simulink library "TurnLightMode_Control"  (R2023a)
settings: Solver=VariableStepAuto  StartTime=0.0  StopTime=10.0  RelTol=1e-3
settings Model: Creator=19856  LastModifiedBy=19856

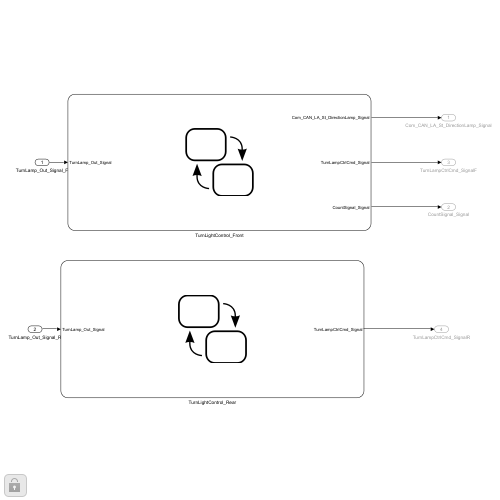
[thumbnail: Simulink's stored preview of the top-level diagram]
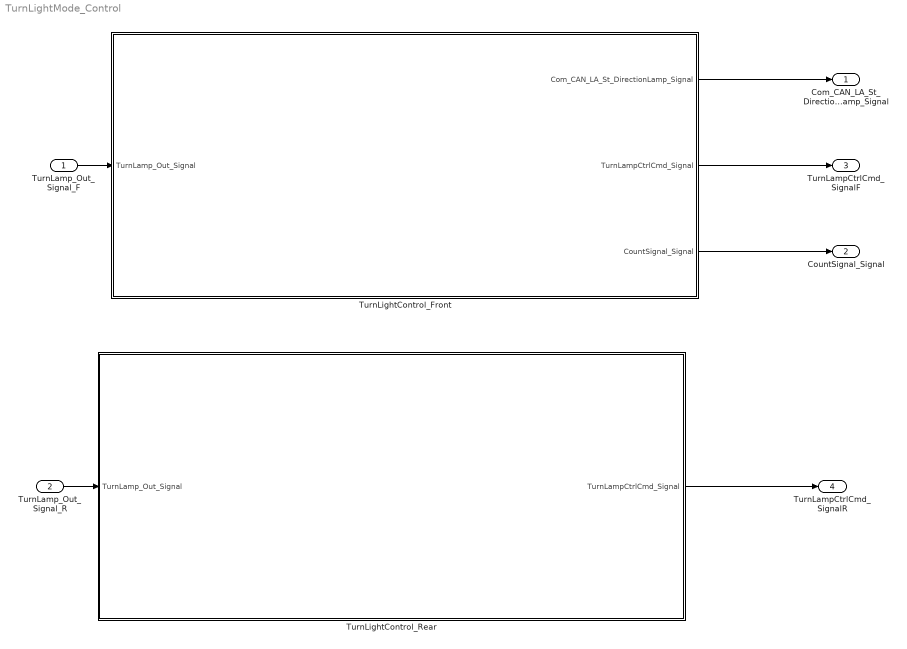
== system TurnLightMode_Control ==
  TurnLamp_Out_Signal_F : Inport
  TurnLamp_Out_Signal_R : Inport  Port=2
  TurnLightControl_Front : Stateflow chart  TreatAsAtomicUnit=on
  TurnLightControl_Rear : Stateflow chart  TreatAsAtomicUnit=on
  Com_CAN_LA_St_DirectionLamp_Signal : Outport
      settings: EnsureOutportIsVirtual=on
  CountSignal_Signal : Outport  Port=2
      settings: EnsureOutportIsVirtual=on
  TurnLampCtrlCmd_SignalF : Outport  Port=3
      settings: EnsureOutportIsVirtual=on
  TurnLampCtrlCmd_SignalR : Outport  Port=4
      settings: EnsureOutportIsVirtual=on
  wires:
  TurnLightControl_Front/2(TurnLampCtrlCmd_Signal) -> TurnLampCtrlCmd_SignalF/1
  TurnLightControl_Front/3(CountSignal_Signal) -> CountSignal_Signal/1
  TurnLamp_Out_Signal_F/1 -> TurnLightControl_Front/1(TurnLamp_Out_Signal)
  TurnLightControl_Front/1(Com_CAN_LA_St_DirectionLamp_Signal) -> Com_CAN_LA_St_DirectionLamp_Signal/1
  TurnLamp_Out_Signal_R/1 -> TurnLightControl_Rear/1(TurnLamp_Out_Signal)
  TurnLightControl_Rear/1(TurnLampCtrlCmd_Signal) -> TurnLampCtrlCmd_SignalR/1

== stateflow chart TurnLightMode_Control/TurnLightControl_Rear ==
  state IDLE
    en:
    TurnLampCtrlCmd_Signal=OFF;
  state LONG
    en:
    CountSignal_Signal=0;
    state OFF
      en:
      TurnLampCtrlCmd_Signal=OFF;
      ex:
      CountSignal_Signal++;
    state ON_
      en:
      TurnLampCtrlCmd_Signal=ON;
    (default) -> LONG.ON_
    LONG.ON_ -> LONG.OFF : [after(400,msec)]
    LONG.OFF -> LONG.ON_ : [after(400,msec)]
  state THREE
    en:
    CountSignal_Signal=0;
    state OFF
      en:
      TurnLampCtrlCmd_Signal=OFF;
      ex:
      CountSignal_Signal++;
    state ON_
      en:
      TurnLampCtrlCmd_Signal=ON;
    (default) -> THREE.ON_
    THREE.ON_ -> THREE.OFF : [after(200,msec)]
    THREE.OFF -> THREE.ON_ : [after(200,msec)]
  (default) -> IDLE
  IDLE -> LONG [order 2] : [TurnLamp_Out_Signal==MODE_LONG||...
      | TurnLamp_Out_Signal==MODE_THREE]
  LONG -> IDLE [order 2] : [TurnLamp_Out_Signal==MODE_THREE&&...
      | CountSignal_Signal==3]
  LONG -> IDLE [order 1] : [hasChangedFrom(TurnLamp_Out_Signal,MODE_LONG)]
  IDLE -> THREE [order 1] : [TurnLamp_Out_Signal==MODE_DOUBLE]
  THREE -> IDLE : [TurnLamp_Out_Signal!=MODE_DOUBLE]
  data: TurnLamp_Out_Signal input uint8; TurnLampCtrlCmd_Signal output uint8; CountSignal_Signal local uint8 =0; MODE_LONG constant uint8 =2; MODE_THREE constant uint8 =1; OFF constant uint8 =0; ON constant uint8 =1; MODE_DOUBLE constant uint8 =3

== stateflow chart TurnLightMode_Control/TurnLightControl_Front ==
  state IDLE
    en:
    TurnLampCtrlCmd_Signal=OFF;
    Com_CAN_LA_St_DirectionLamp_Signal=OFF;
  state NORMAL
    en:
    CountSignal_Signal=0;
    state OFF
      en:
      TurnLampCtrlCmd_Signal=OFF;
      Com_CAN_LA_St_DirectionLamp_Signal=OFF;
      ex:
      CountSignal_Signal++;
    state ON_
      en:
      TurnLampCtrlCmd_Signal=ON;
      Com_CAN_LA_St_DirectionLamp_Signal=ON;
    (default) -> NORMAL.ON_
    NORMAL.ON_ -> NORMAL.OFF : [after(400,msec)]
    NORMAL.OFF -> NORMAL.ON_ : [after(400,msec)]
  state DOUBLE
    en:
    CountSignal_Signal=0;
    state OFF
      en:
      TurnLampCtrlCmd_Signal=OFF;
      Com_CAN_LA_St_DirectionLamp_Signal=OFF;
      ex:
      CountSignal_Signal++;
    state ON_
      en:
      TurnLampCtrlCmd_Signal=ON;
      Com_CAN_LA_St_DirectionLamp_Signal=ON;
    (default) -> DOUBLE.ON_
    DOUBLE.ON_ -> DOUBLE.OFF : [after(200,msec)]
    DOUBLE.OFF -> DOUBLE.ON_ : [after(200,msec)]
  (default) -> IDLE
  IDLE -> NORMAL [order 1] : [TurnLamp_Out_Signal==MODE_LONG||...
      | TurnLamp_Out_Signal==MODE_THREE]
  NORMAL -> IDLE [order 2] : [TurnLamp_Out_Signal==MODE_THREE&&...
      | CountSignal_Signal==3]
  NORMAL -> IDLE [order 1] : [hasChangedFrom(TurnLamp_Out_Signal,MODE_LONG)]
  IDLE -> DOUBLE [order 2] : [TurnLamp_Out_Signal==MODE_DOUBLE]
  DOUBLE -> IDLE : [TurnLamp_Out_Signal!=MODE_DOUBLE]
  data: TurnLamp_Out_Signal input uint8; Com_CAN_LA_St_DirectionLamp_Signal output uint8; TurnLampCtrlCmd_Signal output uint8; CountSignal_Signal output uint8; MODE_LONG constant uint8 =2; MODE_THREE constant uint8 =1; OFF constant uint8 =0; ON constant uint8 =1; MODE_DOUBLE constant uint8 =3
